simulink model "compensadores"  (R2021a)
settings: Solver=VariableStepAuto  StartTime=0.0  StopTime=2.5  RelTol=1e-3
libraries: dspsrcs4 x1, pid_lib x1
settings Model: Creator=Bremdows  LastModifiedBy=Bremdow

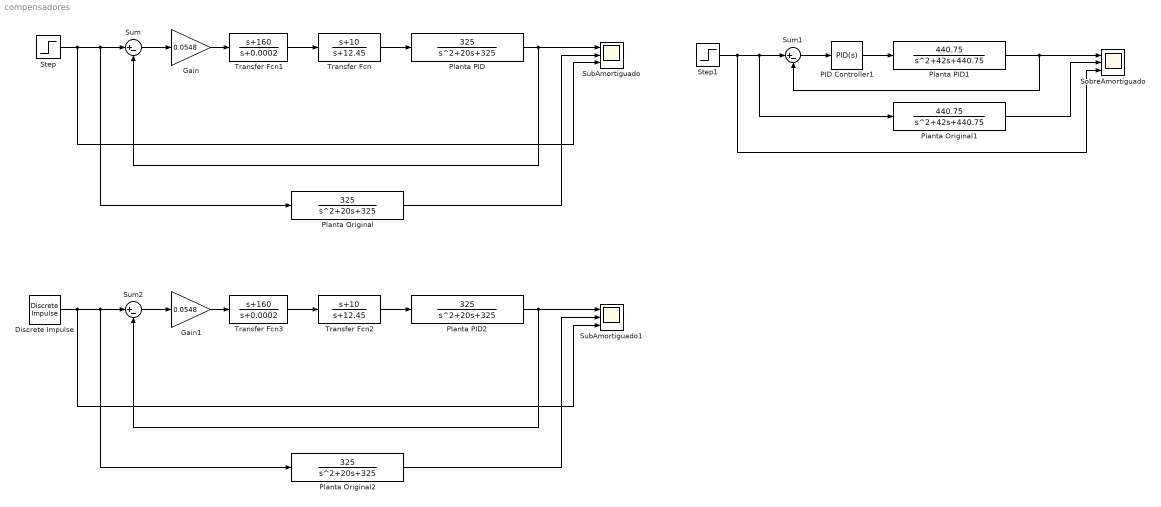
== system compensadores ==
  Discrete Impulse : dspsrcs4/Discrete  Impulse  Delay=0  SampleTime=1  FrameSample=1  OutputFrames=off  dataType=double  isSigned=on  wordLen=16  udDataType=sfix(16)  fracBitsMode=Best precision  numFracBits=15  OutDataTypeStr=double  LastOutDataTypeStr=double
  Gain : Gain  Gain=0.0548
  Gain1 : Gain  Gain=0.0548
  PID Controller1 : pid_lib/PID Controller  Controller=PID  Form=Parallel  TimeDomain=Continuous-time  UseExternalTs=off  SampleTime=-1  IntegratorMethod=Forward Euler  FilterMethod=Forward Euler  ControllerParametersSource=internal  P=6.108  I=64.843  D=0.143  UseFilter=on  N=100  TunerSelectOption=Transfer Function Based (PID Tuner App)  InitialConditionSource=internal  InitialConditionForIntegrator=0  InitialConditionForFilter=0  DifferentiatorICPrevScaledInput=0  ExternalReset=none  TrackingMode=off  Kt=1  LimitOutput=off  SatLimitsSource=internal  UpperSaturationLimit=inf  LowerSaturationLimit=-inf  LinearizeAsGain=on  AntiWindupMode=none  Kb=1  POutMin=[]  POutMax=[]  IOutMin=[]  IOutMax=[]  DOutMin=[]  DOutMax=[]  NOutMin=[]  NOutMax=[]  SumOutMin=[]  SumOutMax=[]  SaturationOutMin=[]  SaturationOutMax=[]  PParamMin=[]  PParamMax=[]  IParamMin=[]  IParamMax=[]  DParamMin=[]  DParamMax=[]  NParamMin=[]  NParamMax=[]  KbParamMin=[]  KbParamMax=[]  KtParamMin=[]  KtParamMax=[]  KbOutMin=[]  KbOutMax=[]  KtOutMin=[]  KtOutMax=[]  IntegratorOutMin=[]  IntegratorOutMax=[]  FilterOutMin=[]  FilterOutMax=[]  SumI1OutMin=[]  SumI1OutMax=[]  SumI2OutMin=[]  SumI2OutMax=[]  SumI3OutMin=[]  SumI3OutMax=[]  SumI4OutMin=[]  SumI4OutMax=[]  SumDOutMin=[]  SumDOutMax=[]  DifferentiatorOutMin=[]  DifferentiatorOutMax=[]  FilterDiffOutCoefMin=[]  FilterDiffOutCoefMax=[]  ReciprocalOutMin=[]  ReciprocalOutMax=[]  SumDenOutMin=[]  SumDenOutMax=[]  SumNumOutMin=[]  SumNumOutMax=[]  DivideOutMin=[]  DivideOutMax=[]  UdiffTsProdOutMin=[]  UdiffTsProdOutMax=[]  NTsProdOutMin=[]  NTsProdOutMax=[]  UintegralTsProdOutMin=[]  UintegralTsProdOutMax=[]  UngainTsProdOutMin=[]  UngainTsProdOutMax=[]  IntegratorContinuousStateAttributes=''  IntegratorStateMustResolveToSignalObject=off  IntegratorRTWStateStorageClass=Auto  FilterContinuousStateAttributes=''  FilterStateMustResolveToSignalObject=off  FilterRTWStateStorageClass=Auto  ParallelPVariant=InternalParameters  IdealPVariant=Disabled  IVariant=InternalParameters  DVariant=InternalParameters  IntegratorVariant=Continuous  SatVariant=Disabled  AWVariant=Passthrough  PCopyVariant=Disabled  TRVariant=Disabled  FdbkBlocksVariant=Forward  IdealPFdbkVariant=Disabled  SatFdbkVariant=Disabled  DerivativeFilterVariant=ContFilter  NVariant=InternalParameters  NCopyVariant=Disabled  FilterICVariant=InternalICsFilter  IntegratorICVariant=InternalICs  ExternalResetVariant=Disabled  TRSumVariant=Passthrough  SumFdbkVariant=Disabled  SumVariant=Sum_PID  TsampFilterVariant=InternalTs  TsampNgainVariant=Passthrough  TsampIntegralVariant=Passthrough  ExternalSaturationOutDataTypeStr=Inherit: Same as second input
  Planta Original : TransferFcn  Numerator=[325]  Denominator=[1 20 325]
  Planta Original1 : TransferFcn  Numerator=[440.75]  Denominator=[1 42 440.75]
  Planta Original2 : TransferFcn  Numerator=[325]  Denominator=[1 20 325]
  Planta PID : TransferFcn  Numerator=[325]  Denominator=[1 20 325]
  Planta PID1 : TransferFcn  Numerator=[440.75]  Denominator=[1 42 440.75]
  Planta PID2 : TransferFcn  Numerator=[325]  Denominator=[1 20 325]
  SobreAmortiguado : Scope  NumInputPorts=3
  Step : Step  Time=0  SampleTime=0
  Step1 : Step  Time=0  SampleTime=0
  SubAmortiguado : Scope  NumInputPorts=3
  SubAmortiguado1 : Scope  NumInputPorts=3
  Sum : Sum  Inputs=|+-
  Sum1 : Sum  Inputs=|+-
  Sum2 : Sum  Inputs=|+-
  Transfer Fcn : TransferFcn  Numerator=[1 10]  Denominator=[1 12.45]
  Transfer Fcn1 : TransferFcn  Numerator=[1 160]  Denominator=[1 0.0002]
  Transfer Fcn2 : TransferFcn  Numerator=[1 10]  Denominator=[1 12.45]
  Transfer Fcn3 : TransferFcn  Numerator=[1 160]  Denominator=[1 0.0002]
  wires:
  Transfer Fcn/1 -> Planta PID/1
  Step/1 -> SubAmortiguado/3, Sum/1, Planta Original/1
  Planta PID/1 -> SubAmortiguado/1, Sum/2
  Planta Original/1 -> SubAmortiguado/2
  Planta Original1/1 -> SobreAmortiguado/2
  Sum1/1 -> PID Controller1/1
  Planta PID1/1 -> SobreAmortiguado/1, Sum1/2
  Step1/1 -> SobreAmortiguado/3, Sum1/1, Planta Original1/1
  PID Controller1/1 -> Planta PID1/1
  Transfer Fcn1/1 -> Transfer Fcn/1
  Gain/1 -> Transfer Fcn1/1
  Sum/1 -> Gain/1
  Gain1/1 -> Transfer Fcn3/1
  Transfer Fcn3/1 -> Transfer Fcn2/1
  Discrete Impulse/1 -> SubAmortiguado1/3, Sum2/1, Planta Original2/1
  Planta Original2/1 -> SubAmortiguado1/2
  Transfer Fcn2/1 -> Planta PID2/1
  Planta PID2/1 -> SubAmortiguado1/1, Sum2/2
  Sum2/1 -> Gain1/1
